simulink model "DynamicModel_BAv01"  (R2022b)
settings: Solver=VariableStepAuto  StartTime=0.0  StopTime=3000  RelTol=1e-3
undefined symbols (not defined in the file): data, getPhysicalConstants, Kp, Ti
libraries: slpidlib x1
settings Model: Creator=giaco  LastModifiedBy=giaco

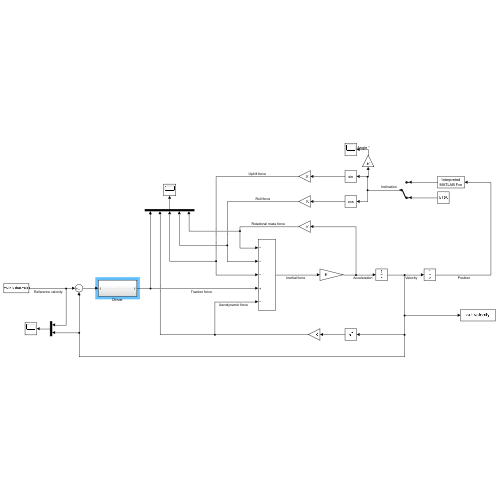
[thumbnail: Simulink's stored preview of the top-level diagram]
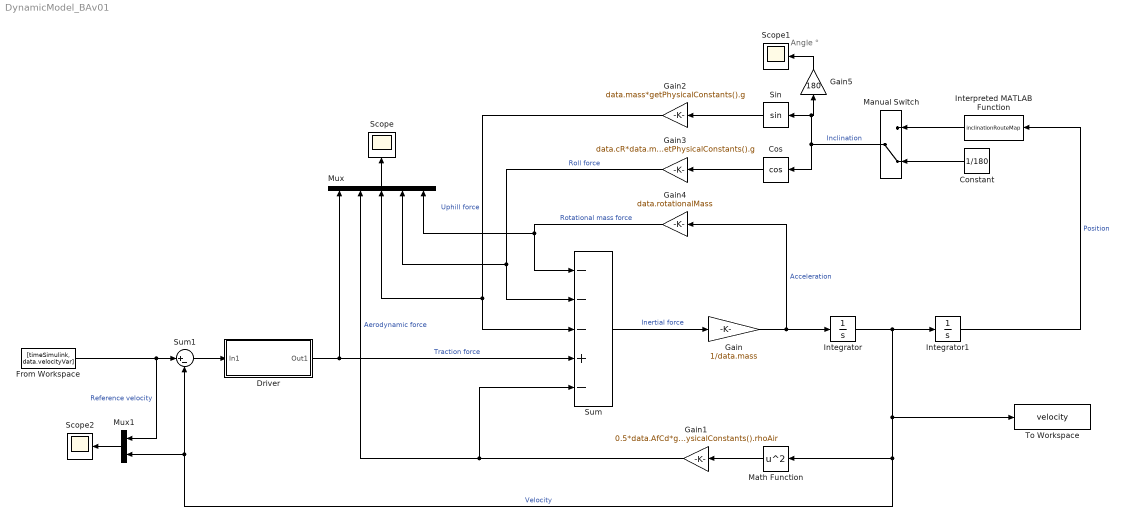
== system DynamicModel_BAv01 ==
  note: Angle °
  Constant : Constant  Value=1/180
  Cos : Trigonometry  Operator=cos
  Driver : Subsystem
  From Workspace : FromWorkspace  VariableName=[timeSimulink, data.velocityVar]
  Gain : Gain  Gain=1/data.mass
  Gain1 : Gain  Gain=0.5*data.AfCd*getPhysicalConstants().rhoAir
  Gain2 : Gain  Gain=data.mass*getPhysicalConstants().g
  Gain3 : Gain  Gain=data.cR*data.mass*getPhysicalConstants().g
  Gain4 : Gain  Gain=data.rotationalMass
  Gain5 : Gain  Gain=180
  Integrator : Integrator
  Integrator1 : Integrator
  Interpreted MATLAB Function : MATLABFcn  MATLABFcn=inclinationRouteMap
  Manual Switch : ManualSwitch  CurrentSetting=0
  Math Function : Math  Operator=square
  Mux : Mux  Inputs=5
  Mux1 : Mux  Inputs=2
  Scope : Scope
  Scope1 : Scope
  Scope2 : Scope
  Sin : Trigonometry
  Sum : Sum  Inputs=---+-
  Sum1 : Sum  Inputs=|+-
  To Workspace : ToWorkspace  VariableName=velocity  SaveFormat=Timeseries  SampleTime=-1
  wires:
  Sum/1 -> Gain/1  "Inertial force"
  Gain/1 -> Gain4/1, Integrator/1  "Acceleration"
  Integrator/1 -> Math Function/1, Sum1/2, Mux1/2, To Workspace/1, Integrator1/1  "Velocity"
  Gain1/1 -> Mux/2, Sum/5  "Aerodynamic force"
  Math Function/1 -> Gain1/1
  From Workspace/1 -> Mux1/1, Sum1/1  "Reference velocity"
  Sum1/1 -> Driver/1(In1)
  Driver/1(Out1) -> Sum/4, Mux/1  "Traction force"
  Manual Switch/1 -> Sin/1, Gain5/1, Cos/1  "Inclination"
  Sin/1 -> Gain2/1
  Gain2/1 -> Mux/3, Sum/3  "Uphill force"
  Cos/1 -> Gain3/1
  Gain3/1 -> Mux/4, Sum/2  "Roll force"
  Gain4/1 -> Mux/5, Sum/1  "Rotational mass force"
  Mux/1 -> Scope/1
  Mux1/1 -> Scope2/1
  Integrator1/1 -> Interpreted MATLAB Function/1  "Position"
  Interpreted MATLAB Function/1 -> Manual Switch/1
  Constant/1 -> Manual Switch/2
  Gain5/1 -> Scope1/1

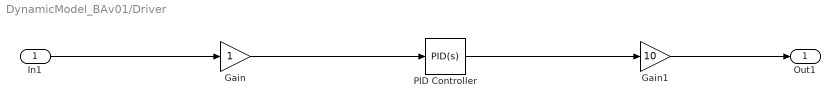
== system DynamicModel_BAv01/Driver ==
  In1 : Inport
  Gain : Gain
  Gain1 : Gain  Gain=10
  PID Controller : slpidlib/PID Controller  Controller=PID  Form=Parallel  TimeDomain=Continuous-time  UseExternalTs=off  SampleTime=-1  IntegratorMethod=Forward Euler  FilterMethod=Forward Euler  ControllerParametersSource=internal  P=Kp  I=Kp/Ti  UseKiTs=off  D=0  N=100  UseFilter=on  TunerSelectOption=Transfer Function Based (PID Tuner App)  InitialConditionSource=internal  InitialConditionForIntegrator=0  InitialConditionForFilter=0  DifferentiatorICPrevScaledInput=0  ExternalReset=none  TrackingMode=off  Kt=1  LimitOutput=off  SatLimitsSource=internal  UpperSaturationLimit=inf  LowerSaturationLimit=-inf  LinearizeAsGain=on  AntiWindupMode=none  Kb=1  LimitIntegrator=off  UpperIntegratorSaturationLimit=inf  LowerIntegratorSaturationLimit=-inf  POutMin=[]  POutMax=[]  IOutMin=[]  IOutMax=[]  DOutMin=[]  DOutMax=[]  NOutMin=[]  NOutMax=[]  SumOutMin=[]  SumOutMax=[]  SaturationOutMin=[]  SaturationOutMax=[]  PParamMin=[]  PParamMax=[]  IParamMin=[]  IParamMax=[]  DParamMin=[]  DParamMax=[]  NParamMin=[]  NParamMax=[]  KbParamMin=[]  KbParamMax=[]  KtParamMin=[]  KtParamMax=[]  KbOutMin=[]  KbOutMax=[]  KtOutMin=[]  KtOutMax=[]  IntegratorOutMin=[]  IntegratorOutMax=[]  FilterOutMin=[]  FilterOutMax=[]  SumI1OutMin=[]  SumI1OutMax=[]  SumI2OutMin=[]  SumI2OutMax=[]  SumI3OutMin=[]  SumI3OutMax=[]  SumI4OutMin=[]  SumI4OutMax=[]  SumDOutMin=[]  SumDOutMax=[]  DifferentiatorOutMin=[]  DifferentiatorOutMax=[]  FilterDiffOutCoefMin=[]  FilterDiffOutCoefMax=[]  ReciprocalOutMin=[]  ReciprocalOutMax=[]  SumDenOutMin=[]  SumDenOutMax=[]  SumNumOutMin=[]  SumNumOutMax=[]  DivideOutMin=[]  DivideOutMax=[]  UdiffTsProdOutMin=[]  UdiffTsProdOutMax=[]  NTsProdOutMin=[]  NTsProdOutMax=[]  UintegralTsProdOutMin=[]  UintegralTsProdOutMax=[]  UngainTsProdOutMin=[]  UngainTsProdOutMax=[]  ClampingZeroOutDataTypeStr=Inherit: Inherit via back propagation  ClampingZeroOutMin=[]  ClampingZeroOutMax=[]  FilterDenConstantOutDataTypeStr=Inherit: Inherit via back propagation  FilterDenConstantOutMin=[]  FilterDenConstantOutMax=[]  PCopyOutDataTypeStr=Inherit: Inherit via back propagation  PCopyOutMin=[]  PCopyOutMax=[]  NCopyOutDataTypeStr=Inherit: Inherit via back propagation  NCopyOutMin=[]  NCopyOutMax=[]  IntegratorContinuousStateAttributes=''  IntegratorStateMustResolveToSignalObject=off  IntegratorRTWStateStorageClass=Auto  FilterContinuousStateAttributes=''  FilterStateMustResolveToSignalObject=off  FilterRTWStateStorageClass=Auto  ParallelPVariant=InternalParameters  IdealPVariant=Disabled  IVariant=InternalParameters  DVariant=InternalParameters  IntegratorVariant=Continuous  SatVariant=Disabled  AWVariant=Passthrough  PCopyVariant=Disabled  TRVariant=Disabled  FdbkBlocksVariant=Forward  IdealPFdbkVariant=Disabled  SatFdbkVariant=Disabled  DerivativeFilterVariant=ContFilter  NVariant=InternalParameters  NCopyVariant=Disabled  FilterICVariant=InternalICsFilter  IntegratorICVariant=InternalICs  ExternalResetVariant=Disabled  TRSumVariant=Passthrough  SumFdbkVariant=Disabled  SumVariant=Sum_PID  TsampFilterVariant=InternalTs  TsampNgainVariant=Passthrough  TsampIntegralVariant=Passthrough  ExternalSaturationOutDataTypeStr=Inherit: Same as second input
  Out1 : Outport
  wires:
  In1/1 -> Gain/1
  PID Controller/1 -> Gain1/1
  Gain/1 -> PID Controller/1
  Gain1/1 -> Out1/1
